simulink model "bh_solenoid_ALL_MODELS"  (R2018a)
settings: Solver=VariableStepAuto  StartTime=0.0  StopTime=3  MaxStep=0.01  RelTol=1e-3  AbsTol=1e-3  EnableMultiTasking=on
CloseFcn:
  | try,close(h1_ssc_solenoid),end
  | clear h1_ssc_solenoid
  | 
  | clear simlog_ssc_solenoid
Description:
  | Solenoid
  | 
  | Copyright 2008-2017 The MathWorks, Inc.
settings Model: Creator=MathWorks  LastModifiedBy=bhorton
settings SolverCC: AutoScaleAbsTol=off
settings DataIOCC: LimitDataPoints=on  SaveFormat=Array
settings OptimizationCC: LifeSpan=inf
settings DebuggingCC: SolverPrmCheckMsg=warning  AllowSymbolicDim=off  SFUnexpectedBacktrackingDiag=warning  SFNoUnconditionalDefaultTransitionDiag=warning  SFExecutionAtInitializationDiag=none
settings HardwareCC: ProdBitPerPointer=32  ProdBitPerSizeT=32  ProdBitPerPtrDiffT=32  ProdLargestAtomicFloat=None  ProdIntDivRoundTo=Undefined  ProdEndianess=Unspecified  ProdWordSize=32  ProdHWDeviceType=32-bit Generic
settings ModelReferenceCC: PropagateSignalLabelsOutOfModel=off
settings CodeAppCC: StateflowObjectComments=on
settings GRTTargetCC: TargetLangStandard=C89/C90 (ANSI)  GeneratePreprocessorConditionals=Disable all
settings ConfigComp: CovMetricSettings=dw  CovHtmlReporting=on  CovSaveCumulativeToWorkspaceVar=on  CovSaveSingleToWorkspaceVar=on  CovExternalEMLEnable=off  CovSFcnEnable=off
settings SimscapeCC: SimscapeLogType=all  SimscapeLogSimulationStatistics=on  SimscapeLogName=simlog_ssc_solenoid  SimscapeLogDataHistory=10000

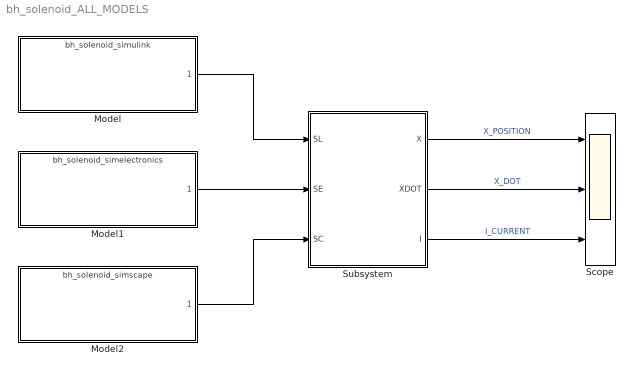
== system bh_solenoid_ALL_MODELS ==
  Model : ModelReference  ModelNameDialog=bh_solenoid_simulink.slx  SimulationMode=Normal  ModelReferenceVersion=1.57
  Model1 : ModelReference  ModelNameDialog=bh_solenoid_simelectronics.slx  SimulationMode=Normal  ModelReferenceVersion=1.36
  Model2 : ModelReference  ModelNameDialog=bh_solenoid_simscape.slx  SimulationMode=Normal  ModelReferenceVersion=1.83
  Scope : Scope  NumInputPorts=3
  Subsystem : Subsystem
  wires:
  Subsystem/1(X) -> Scope/1  "X_POSITION"
  Subsystem/2(XDOT) -> Scope/2  "X_DOT"
  Subsystem/3(I) -> Scope/3  "I_CURRENT"
  Model/1 -> Subsystem/1(SL)
  Model1/1 -> Subsystem/2(SE)
  Model2/1 -> Subsystem/3(SC)

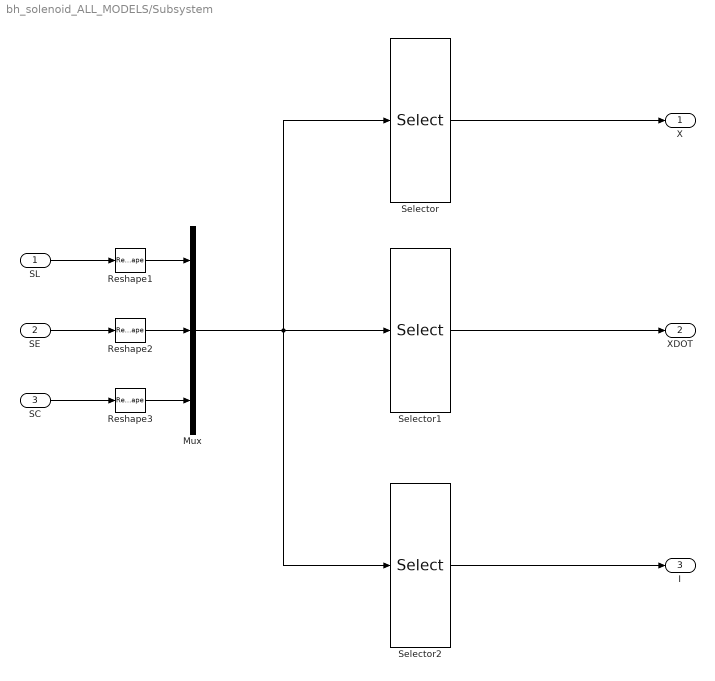
== system bh_solenoid_ALL_MODELS/Subsystem ==
  SL : Inport
  SE : Inport  Port=2
  SC : Inport  Port=3
  Mux : Mux  Inputs=3
  Reshape1 : Reshape  OutputDimensionality=Column vector (2-D)
  Reshape2 : Reshape  OutputDimensionality=Column vector (2-D)
  Reshape3 : Reshape  OutputDimensionality=Column vector (2-D)
  Selector : Selector  InputPortWidth=9  IndexOptions=Index vector (dialog)  Indices=[1 4 7]  OutputSizes=1
  Selector1 : Selector  InputPortWidth=9  IndexOptions=Index vector (dialog)  Indices=1+[1 4 7]  OutputSizes=1
  Selector2 : Selector  InputPortWidth=9  IndexOptions=Index vector (dialog)  Indices=2+[1 4 7]  OutputSizes=1
  X : Outport
  XDOT : Outport  Port=2
  I : Outport  Port=3
  wires:
  SL/1 -> Reshape1/1
  SE/1 -> Reshape2/1
  SC/1 -> Reshape3/1
  Reshape2/1 -> Mux/2
  Reshape1/1 -> Mux/1
  Reshape3/1 -> Mux/3
  Mux/1 -> Selector2/1, Selector/1, Selector1/1
  Selector/1 -> X/1
  Selector1/1 -> XDOT/1
  Selector2/1 -> I/1
